simulink library "Cooling_Tower"  (R2018b)
settings: Solver=ode45  StartTime=0.0  StopTime=10.0  RelTol=1e-3  EnableMultiTasking=on
undefined symbols (not defined in the file): path_carnot
libraries: carnot x11
settings Model: Creator=lena.frank  LastModifiedBy=P41573
settings DataIOCC: LimitDataPoints=on  SaveFormat=Array  SignalLoggingSaveFormat=ModelDataLogs
settings OptimizationCC: ExpressionDepthLimit=2147483647  LifeSpan=inf
settings DebuggingCC: UnderspecifiedInitializationDetection=Classic  MergeDetectMultiDrivingBlocksExec=none  SolverPrmCheckMsg=warning  FcnCallInpInsideContextMsg=warning  StateNameClashWarn=warning  SFUnexpectedBacktrackingDiag=warning  SFNoUnconditionalDefaultTransitionDiag=warning  SFExecutionAtInitializationDiag=none
settings HardwareCC: ProdBitPerPointer=32  ProdBitPerSizeT=32  ProdBitPerPtrDiffT=32  ProdLargestAtomicFloat=None  ProdIntDivRoundTo=Undefined  ProdEndianess=Unspecified  ProdWordSize=32  ProdHWDeviceType=32-bit Generic
settings ModelReferenceCC: PropagateSignalLabelsOutOfModel=off
settings SFSimCC: SimUseLocalCustomCode=off
settings RTWCC: RTWUseLocalCustomCode=off
settings CodeAppCC: StateflowObjectComments=on
settings GRTTargetCC: TargetLangStandard=C89/C90 (ANSI)  GeneratePreprocessorConditionals=Disable all  CombineOutputUpdateFcns=off  GRTInterface=on
settings ConfigComp: CovMetricSettings=dw  CovHtmlReporting=on  CovSaveCumulativeToWorkspaceVar=on  CovSaveSingleToWorkspaceVar=on  CovExternalEMLEnable=off

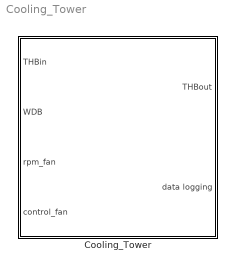
== system Cooling_Tower ==
  Cooling_Tower : Subsystem  mask(Closed Circuit Cooling Tower){}
      mask help:
      | performance data
      | wet-bulb temperature - 15°C ... 24°C
      | rpm fan - 248 1/min (30%) ... 824 1/min (100%)
      | fluid temperature - 26°C ... 44°C
      | fluid flow rate - 1,07 l/s ... 3,03 l/s
      | water/glykol - 0 % ... 100%
      |
      | data logging:
      | wet-bulb temperature....[°C]   (ambient air)
      | rpm fan.........................[%]
      | v_dot fan......................[m³/s]
      | rpm fan.........................[1/min]
      | rel_hum.........................[%]     (ambient air)
      | t_air..............................[°C]    (ambient air)
      | energy ct......................[kJ]    (fan motor + recirculating spray pump)
      | power ct.......................[kW]    (fan motor + recirculating spray pump)
      | water consumption.......[kg]
      | Tnodes.........................[°C]    (inactivity modul)
      | THBout
      mask Help: web(fullfile(path_carnot('help'),'Cooling_Tower.html'),'-helpbrowser')
      mask Display:
      | plot(-20,5,140,80,[20 90 90 20 20],[20 20 70 70 20])
      | plot([30 35],[62 65],[40 35],[62 65],[35 35],[62 65],[80 80],[62 65],[75 80],[62 65],[85 80],[62 65],[57 57],[62 65],[52 57],[62 65],[62 57],[62 65])
      | plot([15 20],[22 22],[15 80],[65 65],[15 15],[22 65],[20 90],[24 24])
      | plot([25 100],[58 58],[25 100],[44 44],[60 25],[51 58],[60 25],[51 44])
      | plot([87 93],[36 36],[87 93],[28 28],[87 82],[36 34],[93 98],[36 34],[87 82],[28 30],[93 98],[28 30],[82 82],[34 30],[98 98],[34 30],[82 95],[34 35],[82 95],[30 29])
      | plot([86 90],[32 32],[90 93],[32 33.5],[90 93],[32 30.5])

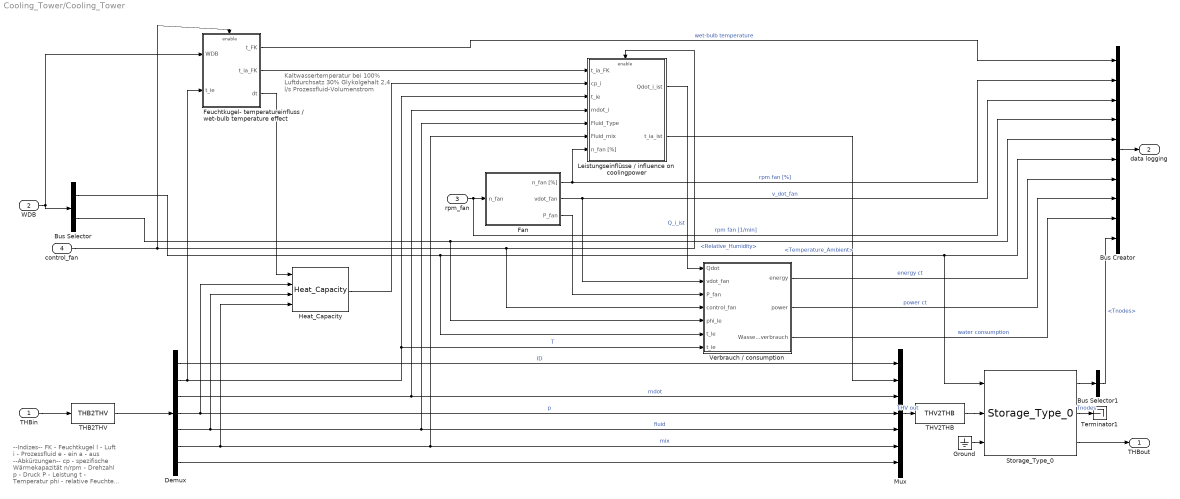
== system Cooling_Tower/Cooling_Tower ==
  note: --Indizes--
      | FK - Feuchtkugel
      | l - Luft
      | i - Prozessfluid
      | e - ein
      | a - aus
      |
      |
      | --Abkürzungen--
      | cp - spezifische Wärmekapazität
      | n/rpm - Drehzahl
      | p - Druck
      | P - Leistung
      | t - Temperatur
      | phi - relative Feuchte
      | x - absolute Feuchte
      | control - Steuersignal
      | mdot - Massenstrom
      | Qdot - Rückkühlleistung
      | vdot - Volumenstrom
  note: Kaltwassertemperatur bei
      | 100% Luftdurchsatz
      | 30% Glykolgehalt
      | 2,4 l/s Prozessfluid-Volumenstrom
  THBin : Inport
  WDB : Inport  Port=2
  rpm_fan : Inport  Port=3
  control_fan : Inport  Port=4
  Bus Creator : BusCreator  Inputs=10
  Bus Selector : BusSelector  OutputSignals=Temperature_Ambient,Relative_Humidity
  Bus Selector1 : BusSelector  OutputSignals=Tnodes
  Demux : Demux  Outputs=[1 1 1 1 1 1 14]
  Fan : Subsystem
  Feuchtkugel- temperatureinfluss / wet-bulb temperature effect : Subsystem
  Ground : Ground
  Heat_Capacity : carnot/Basic/Material_Properties/Heat_Capacity  VariantControl=CarlibClassic  INPUTARGUMENTS=state variables (classic)  DEBUGLEVEL=DEBUGLEVEL  MAXTOTALWARNINGS=inf  MAXCONSECUTIVEWARNINGS=inf  WRITETOFILE=0  FILENAME='errors.txt'
      settings: SourceProductName=Carnot
  Leistungseinflüsse / influence on coolingpower : Subsystem
  Mux : Mux  Inputs=7
  Storage_Type_0 : carnot/Storage/Thermal/Storage_Type_0  t0=20  hgt=0.95493  stgtype=0  mpts=[1 2 3 4 5]  tini=[20 20 20 20 20]  PathName=fullfile(path_carnot('libsl'),'Storage','Thermal','Storage_Type_0','parameter_set')  FileName='<user defined>'  userPath=off  userParam=on  uwall=1  ubot=1  utop=1  axcond=1  volume=0.03  dia=0.2  standing=standing cylinder  nodes=5  mpoints=5  Tsensor=0.5  pipe1inlet=1  pipe1outlet=0  pipe1dia=0.03  heater1start=0.2  heater1end=0.25
      settings: SourceProductName=Carnot
  THB2THV : carnot/Toolbox/THB2THV
      settings: SourceProductName=Carnot
  THV2THB : carnot/Toolbox/THV2THB
      settings: SourceProductName=Carnot
  Terminator1 : Terminator
  Verbrauch / consumption : Subsystem
  THBout : Outport
  data logging : Outport  Port=2
  wires:
  Verbrauch / consumption/1(energy) -> Bus Creator/7  "energy ct"
  Bus Creator/1 -> data logging/1
  WDB/1 -> Bus Selector/1, Feuchtkugel- temperatureinfluss / wet-bulb temperature effect/1(WDB)
  Demux/6 -> Mux/6, Leistungseinflüsse / influence on coolingpower/6(Fluid_mix), Heat_Capacity/4  "mix"
  Verbrauch / consumption/3(Wasserverbrauch) -> Bus Creator/9  "water consumption"
  Bus Selector/1 -> Storage_Type_0/1, Bus Creator/6, Verbrauch / consumption/6(t_le)  "<Temperature_Ambient>"
  Bus Selector/2 -> Bus Creator/5, Verbrauch / consumption/5(phi_le)  "<Relative_Humidity>"
  Fan/1(n_fan [%]) -> Bus Creator/2, Leistungseinflüsse / influence on coolingpower/7(n_fan [%])  "rpm fan [%]"
  Leistungseinflüsse / influence on coolingpower/1(Qdot_i_ist) -> Verbrauch / consumption/1(Qdot)  "Q_i_ist"
  Feuchtkugel- temperatureinfluss / wet-bulb temperature effect/1(t_FK) -> Bus Creator/1  "wet-bulb temperature"
  Demux/1 -> Mux/1  "ID"
  control_fan/1 -> Feuchtkugel- temperatureinfluss / wet-bulb temperature effect/Enable, Leistungseinflüsse / influence on coolingpower/Enable, Verbrauch / consumption/4(control_fan)
  Fan/3(P_fan) -> Verbrauch / consumption/3(P_fan)
  Verbrauch / consumption/2(power) -> Bus Creator/8  "power ct"
  Fan/2(vdot_fan) -> Bus Creator/3, Verbrauch / consumption/2(vdot_fan)  "v_dot_fan"
  Heat_Capacity/1 -> Leistungseinflüsse / influence on coolingpower/2(cp_i)
  Leistungseinflüsse / influence on coolingpower/2(t_ia_ist) -> Mux/2
  Demux/2 -> Verbrauch / consumption/7(t_ie), Leistungseinflüsse / influence on coolingpower/3(t_ie), Feuchtkugel- temperatureinfluss / wet-bulb temperature effect/2(t_ie)  "T"
  Feuchtkugel- temperatureinfluss / wet-bulb temperature effect/2(t_ia_FK) -> Leistungseinflüsse / influence on coolingpower/1(t_ia_FK)
  Feuchtkugel- temperatureinfluss / wet-bulb temperature effect/3(dt) -> Heat_Capacity/1
  rpm_fan/1 -> Bus Creator/4, Fan/1(n_fan)  "rpm fan [1/min]"
  Demux/4 -> Mux/4, Heat_Capacity/2  "p"
  Mux/1 -> THV2THB/1  "THV out"
  Demux/5 -> Leistungseinflüsse / influence on coolingpower/5(Fluid_Type), Mux/5, Heat_Capacity/3  "fluid"
  Demux/7 -> Mux/7
  Demux/3 -> Mux/3, Leistungseinflüsse / influence on coolingpower/4(mdot_i)  "mdot"
  THBin/1 -> THB2THV/1
  Storage_Type_0/3 -> THBout/1
  THV2THB/1 -> Storage_Type_0/2
  THB2THV/1 -> Demux/1
  Storage_Type_0/2 -> Terminator1/1  "Tnodes"
  Storage_Type_0/1 -> Bus Selector1/1
  Bus Selector1/1 -> Bus Creator/10  "<Tnodes>"
  Ground/1 -> Storage_Type_0/3

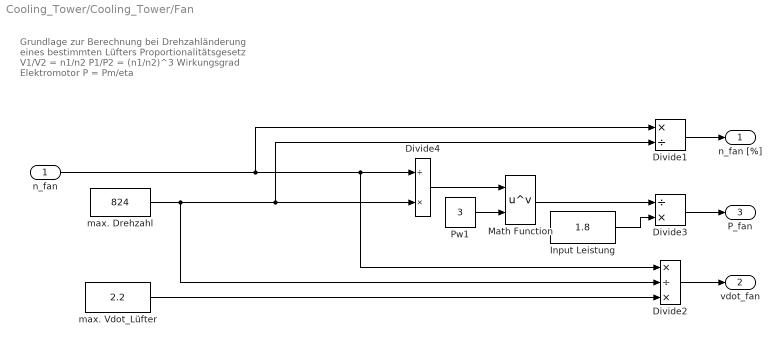
== system Cooling_Tower/Cooling_Tower/Fan ==
  note: Grundlage zur Berechnung
      | bei Drehzahländerung eines bestimmten Lüfters
      |
      | Proportionalitätsgesetz
      | V1/V2 = n1/n2
      | P1/P2 = (n1/n2)^3
      |
      | Wirkungsgrad Elektromotor
      | P = Pm/eta
  n_fan : Inport
  Divide1 : Product  Inputs=*/
  Divide2 : Product  Inputs=*/*
  Divide3 : Product  Inputs=/*
  Divide4 : Product  Inputs=/*
  Input Leistung : Constant  Value=1.8
  Math Function : Math  Operator=pow  SaturateOnIntegerOverflow=on
  Pw1 : Constant  Value=3
  max. Drehzahl : Constant  Value=824
  max. Vdot_Lüfter : Constant  Value=2.2
  n_fan [%] : Outport
  vdot_fan : Outport  Port=2
  P_fan : Outport  Port=3
  wires:
  Pw1/1 -> Math Function/2
  Math Function/1 -> Divide3/1
  Divide4/1 -> Math Function/1
  Divide3/1 -> P_fan/1
  Divide2/1 -> vdot_fan/1
  max. Vdot_Lüfter/1 -> Divide2/3
  Input Leistung/1 -> Divide3/2
  Divide1/1 -> n_fan [%]/1
  max. Drehzahl/1 -> Divide4/2, Divide1/2, Divide2/2
  n_fan/1 -> Divide1/1, Divide4/1, Divide2/1

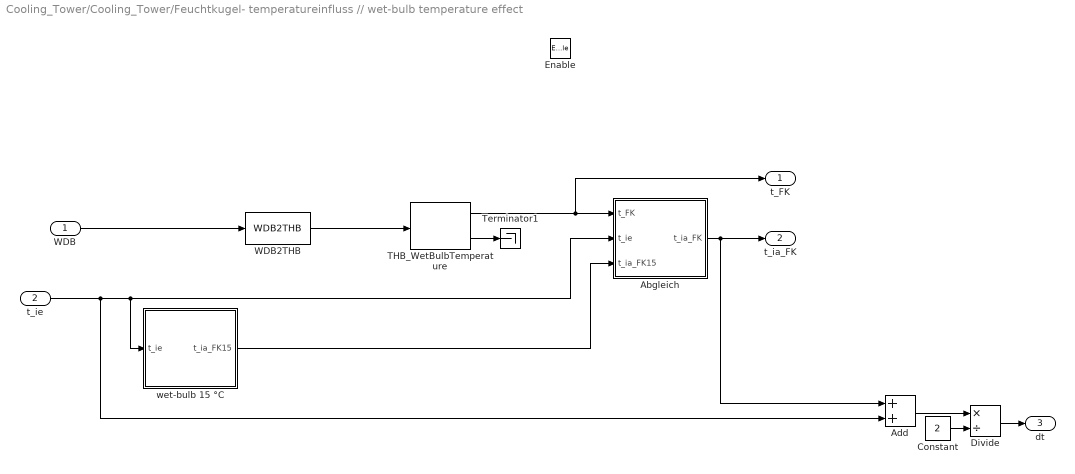
== system Cooling_Tower/Cooling_Tower/Feuchtkugel- temperatureinfluss // wet-bulb temperature effect ==
  WDB : Inport
  t_ie : Inport  Port=2
  Enable : EnablePort
  "Abgleich " : Subsystem
  Add : Sum
  Constant : Constant  Value=2
  Divide : Product  Inputs=*/
  THB_WetBulbTemperature : carnot/Basic/Material_Properties/THB_WetBulbTemperature
      settings: SourceProductName=Carnot
  Terminator1 : Terminator
  WDB2THB : carnot/Weather/WDB2THB  dia=0.2
      settings: SourceProductName=Carnot
  wet-bulb 15 °C : Subsystem
  t_FK : Outport  InitialOutput=0
  t_ia_FK : Outport  Port=2  InitialOutput=0
  dt : Outport  Port=3  InitialOutput=0
  wires:
  Divide/1 -> dt/1
  Constant/1 -> Divide/2
  Add/1 -> Divide/1
  "Abgleich "/1(t_ia_FK) -> t_ia_FK/1, Add/1
  t_ie/1 -> "Abgleich "/2(t_ie), wet-bulb 15 °C/1(t_ie), Add/2
  THB_WetBulbTemperature/1 -> t_FK/1, "Abgleich "/1(t_FK)
  wet-bulb 15 °C/1(t_ia_FK15) -> "Abgleich "/3(t_ia_FK15)
  WDB/1 -> WDB2THB/1
  THB_WetBulbTemperature/2 -> Terminator1/1
  WDB2THB/1 -> THB_WetBulbTemperature/1

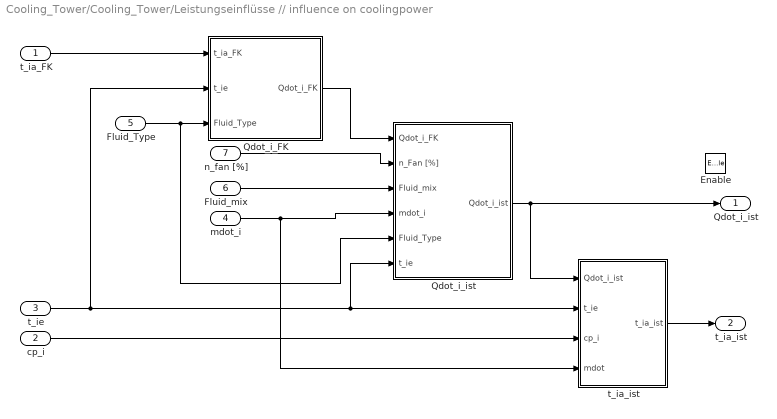
== system Cooling_Tower/Cooling_Tower/Leistungseinflüsse // influence on coolingpower ==
  t_ia_FK : Inport
  cp_i : Inport  Port=2
  t_ie : Inport  Port=3
  mdot_i : Inport  Port=4
  Fluid_Type : Inport  Port=5
  Fluid_mix : Inport  Port=6
  n_fan [%] : Inport  Port=7
  Enable : EnablePort
  Qdot_i_FK : Subsystem
  "Qdot_i_ist " : Subsystem
  "t_ia_ist " : Subsystem
  Qdot_i_ist : Outport  InitialOutput=0
  t_ia_ist : Outport  Port=2  InitialOutput=0
  wires:
  Fluid_mix/1 -> "Qdot_i_ist "/3(Fluid_mix)
  mdot_i/1 -> "t_ia_ist "/4(mdot), "Qdot_i_ist "/4(mdot_i)
  Fluid_Type/1 -> "Qdot_i_ist "/5(Fluid_Type), Qdot_i_FK/3(Fluid_Type)
  cp_i/1 -> "t_ia_ist "/3(cp_i)
  "t_ia_ist "/1(t_ia_ist) -> t_ia_ist/1
  n_fan [%]/1 -> "Qdot_i_ist "/2(n_Fan [%])
  t_ia_FK/1 -> Qdot_i_FK/1(t_ia_FK)
  t_ie/1 -> "Qdot_i_ist "/6(t_ie), "t_ia_ist "/2(t_ie), Qdot_i_FK/2(t_ie)
  Qdot_i_FK/1(Qdot_i_FK) -> "Qdot_i_ist "/1(Qdot_i_FK)
  "Qdot_i_ist "/1(Qdot_i_ist) -> "t_ia_ist "/1(Qdot_i_ist), Qdot_i_ist/1

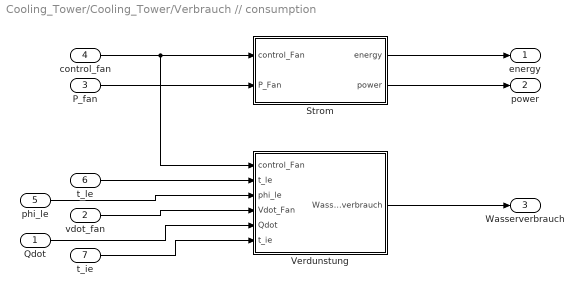
== system Cooling_Tower/Cooling_Tower/Verbrauch // consumption ==
  Qdot : Inport
  vdot_fan : Inport  Port=2
  P_fan : Inport  Port=3
  control_fan : Inport  Port=4
  phi_le : Inport  Port=5
  t_le : Inport  Port=6
  t_ie : Inport  Port=7
  Strom : Subsystem
  Verdunstung : Subsystem
  energy : Outport
  power : Outport  Port=2
  Wasserverbrauch : Outport  Port=3
  wires:
  Strom/1(energy) -> energy/1
  t_ie/1 -> Verdunstung/6(t_ie)
  Qdot/1 -> Verdunstung/5(Qdot)
  vdot_fan/1 -> Verdunstung/4(Vdot_Fan)
  phi_le/1 -> Verdunstung/3(phi_le)
  Verdunstung/1(Wasserverbrauch) -> Wasserverbrauch/1
  t_le/1 -> Verdunstung/2(t_le)
  Strom/2(power) -> power/1
  P_fan/1 -> Strom/2(P_Fan)
  control_fan/1 -> Verdunstung/1(control_Fan), Strom/1(control_Fan)

== system Cooling_Tower/Cooling_Tower/Feuchtkugel- temperatureinfluss // wet-bulb temperature effect/Abgleich  ==
  note: Durch den Abgleich der vorliegenden Datensätze
      | wierd die Annahme getroffen
      | das bei einer reduzierung der Feuchtkugeltemp um 1K
      |  sich die Kaltwassertemp um 0.27K sinkt.
      |
      | y = ((t_FK-15)*0.27)+t_ia_100
      |
      | Ab eine Eintritstemperatur von 41 °C wierd mit
      | dem Faktor 0,25 K gerechnet.
      |
      | y = ((t_FK-15)*0.25)+t_ia_100
  t_FK : Inport
  t_ie : Inport  Port=2
  t_ia_FK15 : Inport  Port=3
  Embedded MATLAB Function : MATLAB Function  TreatAsAtomicUnit=on
  t_ia_FK : Outport
  wires:
  t_ie/1 -> Embedded MATLAB Function/3(t_ie)
  t_ia_FK15/1 -> Embedded MATLAB Function/2(t_ia_fk15)
  t_FK/1 -> Embedded MATLAB Function/1(t_fk)
  Embedded MATLAB Function/1(y) -> t_ia_FK/1

== system Cooling_Tower/Cooling_Tower/Feuchtkugel- temperatureinfluss // wet-bulb temperature effect/wet-bulb 15 °C ==
  t_ie : Inport
  Lookup Table : Lookup  InputValues=[26 28 30 32 34 36 38 40 42 44 79.2]  Table=[22.6 23.9 25.2 26.4 27.7 28.9 30.1 31.2 32.4 33.5 49.25]
  t_ia_FK15 : Outport
  wires:
  Lookup Table/1 -> t_ia_FK15/1
  t_ie/1 -> Lookup Table/1

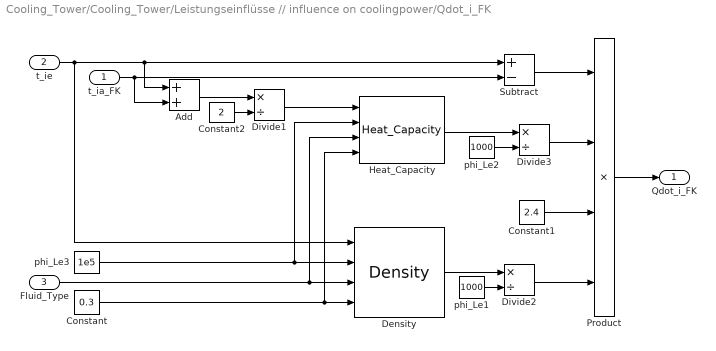
== system Cooling_Tower/Cooling_Tower/Leistungseinflüsse // influence on coolingpower/Qdot_i_FK ==
  t_ia_FK : Inport
  t_ie : Inport  Port=2
  Fluid_Type : Inport  Port=3
  Add : Sum
  Constant : Constant  Value=0.3
  Constant1 : Constant  Value=2.4
  Constant2 : Constant  Value=2
  Density : carnot/Basic/Material_Properties/Density  VariantControl=CarlibClassic  INPUTARGUMENTS=state variables (classic)  DEBUGLEVEL=DEBUGLEVEL  MAXTOTALWARNINGS=inf  MAXCONSECUTIVEWARNINGS=inf  WRITETOFILE=0  FILENAME='errors.txt'
      settings: SourceProductName=Carnot
  Divide1 : Product  Inputs=*/
  Divide2 : Product  Inputs=*/
  Divide3 : Product  Inputs=*/
  Heat_Capacity : carnot/Basic/Material_Properties/Heat_Capacity  VariantControl=CarlibClassic  INPUTARGUMENTS=state variables (classic)  DEBUGLEVEL=DEBUGLEVEL  MAXTOTALWARNINGS=inf  MAXCONSECUTIVEWARNINGS=inf  WRITETOFILE=0  FILENAME='errors.txt'
      settings: SourceProductName=Carnot
  Product : Product  Inputs=4  RndMeth=Zero
  Subtract : Sum  Inputs=+-
  phi_Le1 : Constant  Value=1000
  phi_Le2 : Constant  Value=1000
  phi_Le3 : Constant  Value=1e5
  Qdot_i_FK : Outport
  wires:
  Divide3/1 -> Product/2
  phi_Le2/1 -> Divide3/2
  Add/1 -> Divide1/1
  Divide1/1 -> Heat_Capacity/1
  Constant2/1 -> Divide1/2
  Heat_Capacity/1 -> Divide3/1
  Constant1/1 -> Product/3
  Divide2/1 -> Product/4
  phi_Le1/1 -> Divide2/2
  Fluid_Type/1 -> Density/3, Heat_Capacity/3
  phi_Le3/1 -> Density/2, Heat_Capacity/2
  Density/1 -> Divide2/1
  Constant/1 -> Density/4, Heat_Capacity/4
  t_ie/1 -> Add/1, Subtract/1, Density/1
  Subtract/1 -> Product/1
  Product/1 -> Qdot_i_FK/1
  t_ia_FK/1 -> Add/2, Subtract/2

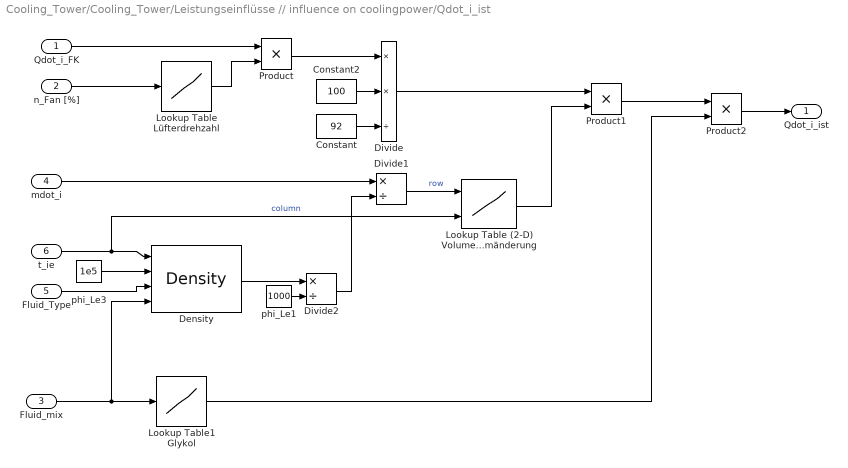
== system Cooling_Tower/Cooling_Tower/Leistungseinflüsse // influence on coolingpower/Qdot_i_ist  ==
  Qdot_i_FK : Inport
  n_Fan [%] : Inport  Port=2
  Fluid_mix : Inport  Port=3
  mdot_i : Inport  Port=4
  Fluid_Type : Inport  Port=5
  t_ie : Inport  Port=6
  Constant : Constant  Value=92
  Constant2 : Constant  Value=100
  Density : carnot/Basic/Material_Properties/Density  VariantControl=CarlibClassic  INPUTARGUMENTS=state variables (classic)  DEBUGLEVEL=DEBUGLEVEL  MAXTOTALWARNINGS=inf  MAXCONSECUTIVEWARNINGS=inf  WRITETOFILE=0  FILENAME='errors.txt'
      settings: SourceProductName=Carnot
  Divide : Product  Inputs=**/
  Divide1 : Product  Inputs=*/
  Divide2 : Product  Inputs=*/
  Lookup Table (2-D) Volumenstromänderung : Lookup2D  RowIndex=[1.07 1.77 2.4 2.65 3.03]  ColumnIndex=[25 30 35 40 45 50 55 60 65]  Table=[0.7248 0.7054 0.6860 0.6666 0.6472 0.6278 0.6084 0.5890 0.5696; 0.9493 0.9294 0.9096 0.8897 0.8698 0.8500 0.8301 0.8103 0.7904; 1 1 1 1 1 1 1 1 1; 1.1191 1.1295 1.0956 1.0674 1.0450 1.0284 1.0175 1.0123 1.0129; 1.2370 1.1910 1.1526 1.1219 1.0988 1.0833 1.0754 1.0752 1.0826]
  Lookup Table Lüfterdrehzahl : Lookup  InputValues=[0 0.2 0.3 0.5 0.7 0.9 1]  Table=[0 0.37 0.482 0.625 0.786 0.928 1]
  Lookup Table1 Glykol : Lookup  InputValues=[0 0.1 0.2 0.3 0.4 0.5 0.6 0.7 0.8 0.9 1]  Table=[1 0.98 0.95 0.92 0.875 0.83 0.78 0.73 0.68 0.63 0.57]
  Product : Product  RndMeth=Zero
  Product1 : Product  RndMeth=Zero
  Product2 : Product  RndMeth=Zero
  phi_Le1 : Constant  Value=1000
  phi_Le3 : Constant  Value=1e5
  Qdot_i_ist : Outport
  wires:
  Constant2/1 -> Divide/2
  Lookup Table (2-D) Volumenstromänderung/1 -> Product1/2
  Divide1/1 -> Lookup Table (2-D) Volumenstromänderung/1  "row"
  t_ie/1 -> Lookup Table (2-D) Volumenstromänderung/2, Density/1  "column"
  Divide2/1 -> Divide1/2
  phi_Le1/1 -> Divide2/2
  Fluid_Type/1 -> Density/3
  phi_Le3/1 -> Density/2
  Density/1 -> Divide2/1
  Product2/1 -> Qdot_i_ist/1
  mdot_i/1 -> Divide1/1
  Constant/1 -> Divide/3
  Divide/1 -> Product1/1
  Fluid_mix/1 -> Lookup Table1 Glykol/1, Density/4
  Lookup Table1 Glykol/1 -> Product2/2
  Product1/1 -> Product2/1
  Product/1 -> Divide/1
  Qdot_i_FK/1 -> Product/1
  Lookup Table Lüfterdrehzahl/1 -> Product/2
  n_Fan [%]/1 -> Lookup Table Lüfterdrehzahl/1

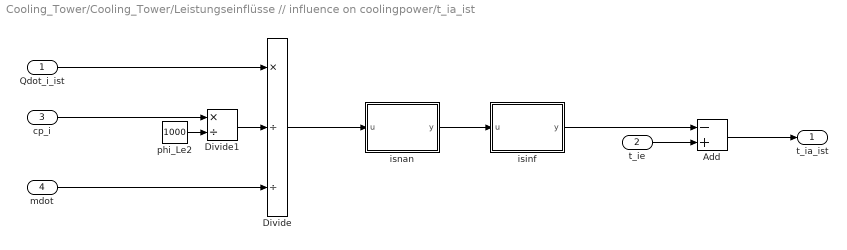
== system Cooling_Tower/Cooling_Tower/Leistungseinflüsse // influence on coolingpower/t_ia_ist  ==
  Qdot_i_ist : Inport
  t_ie : Inport  Port=2
  cp_i : Inport  Port=3
  mdot : Inport  Port=4
  Add : Sum  Inputs=-+
  Divide : Product  Inputs=*//
  Divide1 : Product  Inputs=*/
  isinf : MATLAB Function  TreatAsAtomicUnit=on
  isnan : MATLAB Function  TreatAsAtomicUnit=on
  phi_Le2 : Constant  Value=1000
  t_ia_ist : Outport
  wires:
  isinf/1(y) -> Add/1
  mdot/1 -> Divide/3
  Divide1/1 -> Divide/2
  phi_Le2/1 -> Divide1/2
  isnan/1(y) -> isinf/1(u)
  cp_i/1 -> Divide1/1
  Divide/1 -> isnan/1(u)
  t_ie/1 -> Add/2
  Qdot_i_ist/1 -> Divide/1
  Add/1 -> t_ia_ist/1

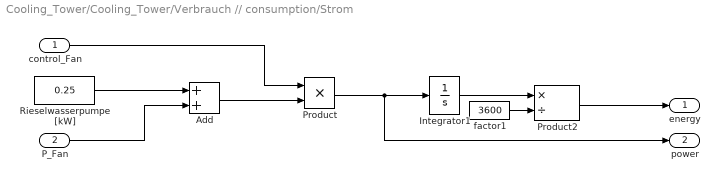
== system Cooling_Tower/Cooling_Tower/Verbrauch // consumption/Strom ==
  control_Fan : Inport
  P_Fan : Inport  Port=2
  Add : Sum
  Integrator1 : Integrator
  Product : Product  RndMeth=Zero
  Product2 : Product  Inputs=*/  SaturateOnIntegerOverflow=on  RndMeth=Zero  InputSameDT=on  OutDataTypeStr=Inherit: Same as first input
  Rieselwasserpumpe [kW] : Constant  Value=0.25
  factor1 : Constant  Value=3600
  energy : Outport
  power : Outport  Port=2
  wires:
  Product2/1 -> energy/1
  factor1/1 -> Product2/2
  Integrator1/1 -> Product2/1
  P_Fan/1 -> Add/2
  Add/1 -> Product/2
  control_Fan/1 -> Product/1
  Product/1 -> Integrator1/1, power/1
  Rieselwasserpumpe [kW]/1 -> Add/1

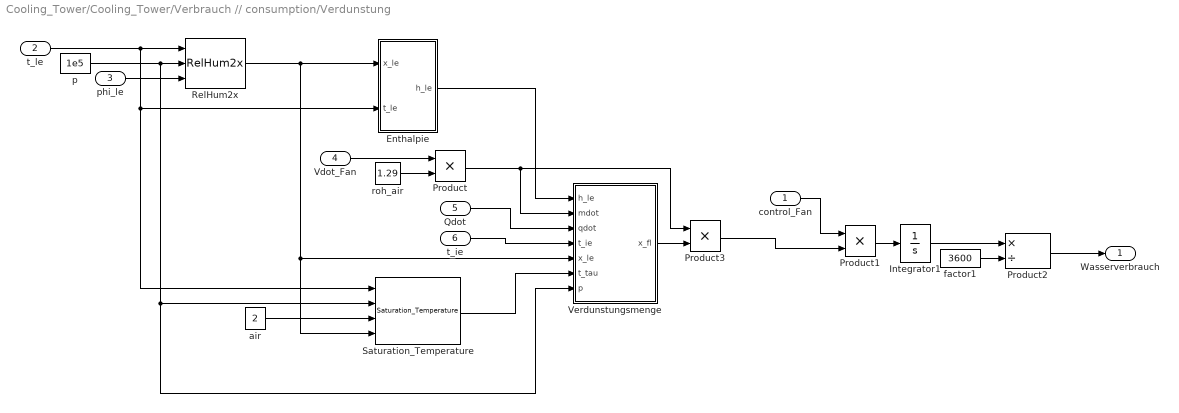
== system Cooling_Tower/Cooling_Tower/Verbrauch // consumption/Verdunstung ==
  control_Fan : Inport
  t_le : Inport  Port=2
  phi_le : Inport  Port=3
  Vdot_Fan : Inport  Port=4
  Qdot : Inport  Port=5
  t_ie : Inport  Port=6
  "Enthalpie " : Subsystem
  Integrator1 : Integrator
  Product : Product  RndMeth=Zero
  Product1 : Product  RndMeth=Zero
  Product2 : Product  Inputs=*/  SaturateOnIntegerOverflow=on  RndMeth=Zero  InputSameDT=on  OutDataTypeStr=Inherit: Same as first input
  Product3 : Product  RndMeth=Zero
  RelHum2x : carnot/Basic/Material_Properties/RelHum2x
      settings: SourceProductName=Carnot
  Saturation_Temperature : carnot/Basic/Material_Properties/Saturation_Temperature  VariantControl=CarlibClassic  INPUTARGUMENTS=state variables (classic)  DEBUGLEVEL=WARNINGLEVEL  MAXTOTALMESSAGES=inf  MAXCONSECUTIVEMESSAGES=inf  WRITETOFILE=0  FILENAME='errors.txt'
      settings: SourceProductName=Carnot
  Verdunstungsmenge : MATLAB Function  TreatAsAtomicUnit=on
  air : Constant  Value=2
  factor1 : Constant  Value=3600
  p : Constant  Value=1e5
  roh_air : Constant  Value=1.29
  Wasserverbrauch : Outport
  wires:
  Verdunstungsmenge/1(x_fl) -> Product3/2
  t_ie/1 -> Verdunstungsmenge/4(t_ie)
  Product/1 -> Product3/1, Verdunstungsmenge/2(mdot)
  Product3/1 -> Product1/2
  control_Fan/1 -> Product1/1
  Product1/1 -> Integrator1/1
  Product2/1 -> Wasserverbrauch/1
  factor1/1 -> Product2/2
  Integrator1/1 -> Product2/1
  air/1 -> Saturation_Temperature/3
  Saturation_Temperature/1 -> Verdunstungsmenge/6(t_tau)
  Qdot/1 -> Verdunstungsmenge/3(qdot)
  RelHum2x/1 -> Verdunstungsmenge/5(x_le), Saturation_Temperature/4, "Enthalpie "/1(x_le)
  "Enthalpie "/1(h_le) -> Verdunstungsmenge/1(h_le)
  roh_air/1 -> Product/2
  Vdot_Fan/1 -> Product/1
  phi_le/1 -> RelHum2x/3
  p/1 -> Verdunstungsmenge/7(p), Saturation_Temperature/2, RelHum2x/2
  t_le/1 -> "Enthalpie "/2(t_le), Saturation_Temperature/1, RelHum2x/1

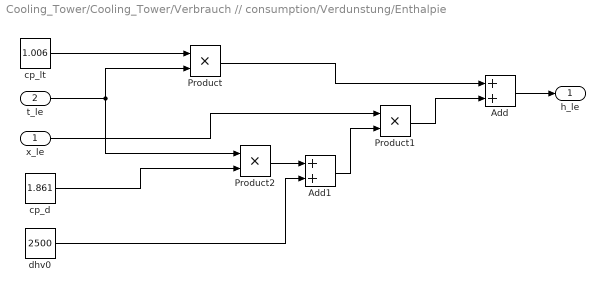
== system Cooling_Tower/Cooling_Tower/Verbrauch // consumption/Verdunstung/Enthalpie  ==
  x_le : Inport
  t_le : Inport  Port=2
  Add : Sum
  Add1 : Sum
  Product : Product  RndMeth=Zero
  Product1 : Product  RndMeth=Zero
  Product2 : Product  RndMeth=Zero
  cp_d : Constant  Value=1.861
  cp_lt : Constant  Value=1.006
  dhv0 : Constant  Value=2500
  h_le : Outport
  wires:
  dhv0/1 -> Add1/2
  Product2/1 -> Add1/1
  Add1/1 -> Product1/2
  cp_d/1 -> Product2/2
  x_le/1 -> Product1/1
  Product1/1 -> Add/2
  Product/1 -> Add/1
  t_le/1 -> Product2/1, Product/2
  cp_lt/1 -> Product/1
  Add/1 -> h_le/1

== matlab function Cooling_Tower/Feuchtkugel- temperatureinfluss // wet-bulb temperature effect/Abgleich /Embedded MATLAB Function ==
  data: t_fk input; y output; t_ia_fk15 input; t_ie input
%Festlegung der Eingänge
function y = fcn(t_fk, t_ia_fk15, t_ie)

%Änderung des Faktors
if t_ie < 41
    
    y = ((t_fk-15)*0.27)+t_ia_fk15;
    
else
    
    y = ((t_fk-15)*0.25)+t_ia_fk15;
    
end

== matlab function Cooling_Tower/Leistungseinflüsse // influence on coolingpower/t_ia_ist /isinf ==
  data: u input; y output

function y = fcn(u)

%Verhindert die Fehlerausgabe bei Teilen mit dem Wert 0 
%Dieser Zustand tritt ein wenn der Volumenstrom 0 l/s gesetzt wird.

v = isinf (u);

if v == 0
    
    y = u;

else 
    
    y = 0;
    
end

== matlab function Cooling_Tower/Leistungseinflüsse // influence on coolingpower/t_ia_ist /isnan ==
  data: u input; y output

function y = fcn(u)

%Verhindert die Fehlerausgabe bei Teilen durch den Wert 0 
%Dieser Zustand tritt ein wenn der Volumenstrom 0 l/s gesetzt wird.

v = isnan (u);

if v == 0
    
    y = u;

else 
    
    y = 0;
    
end

== matlab function Cooling_Tower/Verbrauch // consumption/Verdunstung/Verdunstungsmenge ==
  data: h_le input; mdot input; x_fl output; qdot input; t_ie input; x_le input; t_tau input; p input
function x_fl = fcn(h_le, mdot, qdot, t_ie, x_le, t_tau, p)

cp_lt = 1.006;
cp_d = 1.861;
cp_w = 4.19;
dhv0 = 2500;
tmax = t_ie;
tmin = t_tau;
t_zw = 15;
phi_luftaus = 100;
m = 1;


% Vorbedingung qdot muss positiv sein um eine Verdunstung zu gewährleisten ansonsten ist es ein Kondensation
if qdot < 0
    
    x_luftaus = 0;
    
else
    % Luftaustrittstemperaturberechnung, Halbierungsverfahren
        t_luftaus = (tmax+tmin)/2;
    
    % Absolute Feuchte-Berechnung Lufteintritt
        ps_luftaus = 611*exp((-1.91275)*10^(-4)+7.258*10^(-2)*t_luftaus-2.939*10^(-4)*t_luftaus^2+9.841*10^(-7)*t_luftaus^3-1.92*10^(-9)*t_luftaus^4);
        x_luftaus = (0.622*(phi_luftaus/100)*ps_luftaus)/(p-(phi_luftaus/100)*ps_luftaus);

    % Enthalpie Luftaustritt mit dem schon berechneten Qpkt
        h_la = qdot/mdot + (x_luftaus-x_le)*cp_w*t_zw + h_le;
    
    % Austrittstemperatur 
        tlab = (h_la - x_luftaus*dhv0)/(cp_lt + x_luftaus*cp_d);

    % Beginn der Schleife 
    % (t_luftaus - tlab) < 0,001 und > -0,001 ist die Austrittstemperatur gefunden
    %  t_luftaus < tlab  tmin = t_luftaus
    %  t_luftaus > tlab  tmax = t_luftaus
        while (t_luftaus - tlab)>0.001 || (t_luftaus - tlab) < -0.001 && m < 30
    
            if t_luftaus < tlab
        
                tmin = t_luftaus;
    
            else
        
                tmax = t_luftaus;
    
            end
    
            % Luftaustrittstemperaturberechnung, Halbierungsverfahren
                t_luftaus = (tmax+tmin)/2;
    
            % Absolute Feuchte-Berechnung Lufteintritt
                ps_luftaus = 611*exp((-1.91275)*10^(-4)+7.258*10^(-2)*t_luftaus-2.939*10^(-4)*t_luftaus^2+9.841*10^(-7)*t_luftaus^3-1.92*10^(-9)*t_luftaus^4);
                x_luftaus = (0.622*(phi_luftaus/100)*ps_luftaus)/(p-(phi_luftaus/100)*ps_luftaus);
        
            % Enthalpie Luftaustritt mit dem schon berechneten Qpkt
                h_la = qdot/mdot + (x_luftaus-x_le)*cp_w*t_zw + h_le;
        
            % Austrittstemperatur 
                tlab = (h_la - x_luftaus*dhv0)/(cp_lt + x_luftaus*cp_d);
        
            % Schleifenzähler
                m = m + 1;
    
        end

end

x_fl = x_luftaus-x_le;
